simulink model "part2_2"  (R2020b)
settings: Solver=VariableStepAuto  StartTime=0.0  StopTime=400  RelTol=1e-3
settings Model: Creator=lipeisoh  LastModifiedBy=lipeisoh

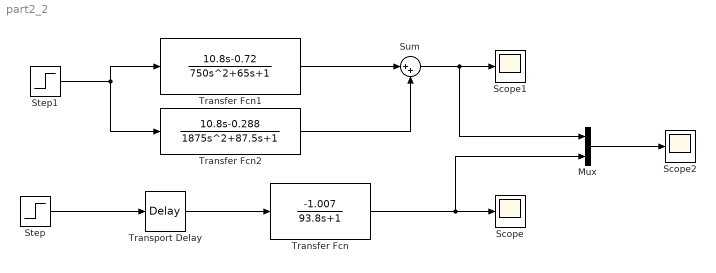
== system part2_2 ==
  Mux : Mux  Inputs=2
  Scope : Scope
  Scope1 : Scope
  Scope2 : Scope
  Step : Step  Time=0  SampleTime=0
  Step1 : Step  Time=0  SampleTime=0
  Sum : Sum  Inputs=|++
  Transfer Fcn : TransferFcn  Numerator=[-1.007]  Denominator=[93.8 1]
  Transfer Fcn1 : TransferFcn  Numerator=[10.8 -0.72]  Denominator=[750 65 1]
  Transfer Fcn2 : TransferFcn  Numerator=[10.8 -0.288]  Denominator=[1875 87.5 1]
  Transport Delay : TransportDelay  DelayTime=26
  wires:
  Transfer Fcn/1 -> Mux/2, Scope/1
  Step/1 -> Transport Delay/1
  Transport Delay/1 -> Transfer Fcn/1
  Step1/1 -> Transfer Fcn1/1, Transfer Fcn2/1
  Transfer Fcn1/1 -> Sum/1
  Transfer Fcn2/1 -> Sum/2
  Sum/1 -> Mux/1, Scope1/1
  Mux/1 -> Scope2/1
